simulink model "lab2"  (R2018b)
settings: Solver=ode45  StartTime=0.0  StopTime=200  RelTol=1e-3
values from neighbouring files (symbols this model uses):
  b = a    [laborator4.m]
undefined symbols (not defined in the file or in its folder): g, m
settings Model: Creator=FetCatz  LastModifiedBy=FetCatz
settings SolverCC: ZeroCrossControl=DisableAll  AutoInsertRateTranBlk=on

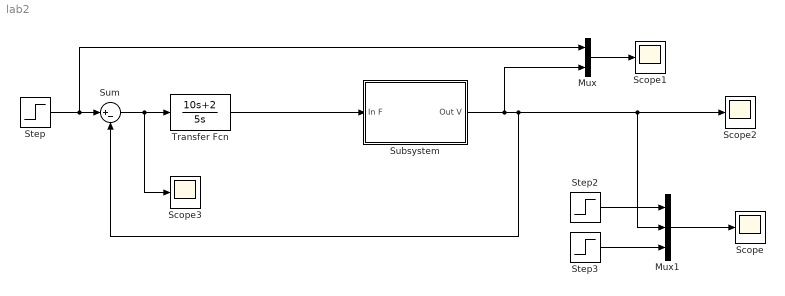
== system lab2 ==
  Mux : Mux  Inputs=2
  Mux1 : Mux  Inputs=3
  Scope{,1..3} (4 alike) : Scope
  Step : Step  Time=0  SampleTime=0
  Step2 : Step  Time=0  SampleTime=0
  Step3 : Step  Time=0  SampleTime=0
  Subsystem : Subsystem
  Sum : Sum  Inputs=|+-
  Transfer Fcn : TransferFcn  Numerator=[10 2]  Denominator=[5 0]
  wires:
  Subsystem/1("Out V ") -> Mux1/2, Scope2/1, Sum/2, Mux/2
  Mux1/1 -> Scope/1
  Mux/1 -> Scope1/1
  Step/1 -> Sum/1, Mux/1
  Step3/1 -> Mux1/3
  Sum/1 -> Scope3/1, Transfer Fcn/1
  Transfer Fcn/1 -> Subsystem/1(In F)
  Step2/1 -> Mux1/1

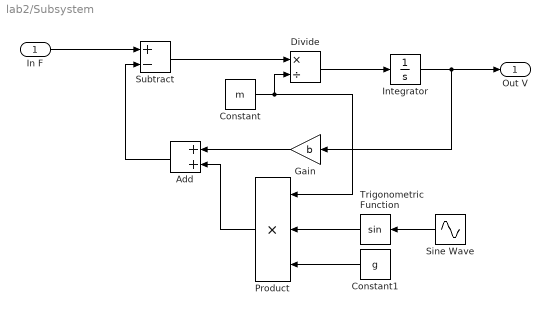
== system lab2/Subsystem ==
  In F : Inport
  Add : Sum
  Constant : Constant  Value=m
  Constant1 : Constant  Value=g
  Divide : Product  Inputs=*/
  Gain : Gain  Gain=b
  Integrator : Integrator
  Product : Product  Inputs=3
  Sine Wave : Sin  Amplitude=0.9  Frequency=0.09  Phase=1  SampleTime=0
  Subtract : Sum  Inputs=+-
  Trigonometric Function : Trigonometry
  "Out V " : Outport
  wires:
  In F/1 -> Subtract/1
  Integrator/1 -> "Out V "/1, Gain/1
  Divide/1 -> Integrator/1
  Subtract/1 -> Divide/1
  Constant/1 -> Product/1, Divide/2
  Gain/1 -> Add/1
  Add/1 -> Subtract/2
  Product/1 -> Add/2
  Trigonometric Function/1 -> Product/2
  Constant1/1 -> Product/3
  Sine Wave/1 -> Trigonometric Function/1
